simulink model "rate_limited_systems"  (R2021a)
settings: Solver=VariableStepAuto  StartTime=0.0  StopTime=10.0  RelTol=1e-3
settings Model: Creator=dimpa  LastModifiedBy=dimpa

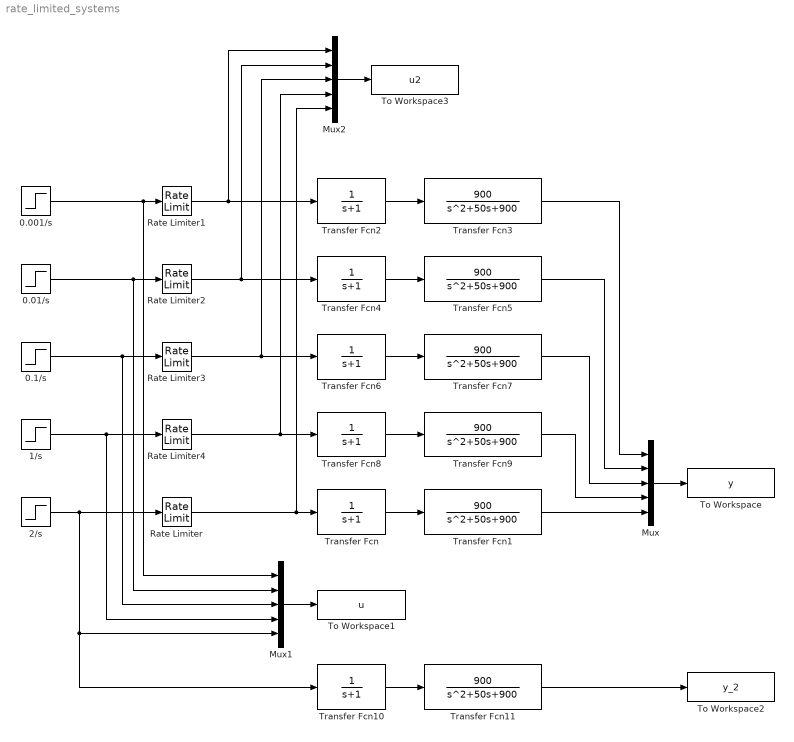
== system rate_limited_systems ==
  0.001/s : Step  After=0.001  SampleTime=0
  0.01/s : Step  After=0.01  SampleTime=0
  0.1/s : Step  After=0.1  SampleTime=0
  1/s : Step  SampleTime=0
  2/s : Step  After=2  SampleTime=0
  Mux : Mux  Inputs=5
  Mux1 : Mux  Inputs=5
  Mux2 : Mux  Inputs=5
  Rate Limiter{,1..4} (5 alike) : RateLimiter  RisingSlewLimit=0.3  SampleTimeMode=inherited
  To Workspace : ToWorkspace  VariableName=y  SaveFormat=Timeseries  SampleTime=-1
  To Workspace1 : ToWorkspace  VariableName=u  SaveFormat=Timeseries  SampleTime=-1
  To Workspace2 : ToWorkspace  VariableName=y_2  SaveFormat=Timeseries  SampleTime=-1
  To Workspace3 : ToWorkspace  VariableName=u2  SaveFormat=Timeseries  SampleTime=-1
  Transfer Fcn{,2,4,6,8,10} (6 alike) : TransferFcn  Denominator=[1 1]
  Transfer Fcn{1,3,5,7,9,11} (6 alike) : TransferFcn  Numerator=[900]  Denominator=[1 50 900]
  wires:
  0.001/s/1 -> Mux1/1, Rate Limiter1/1
  0.01/s/1 -> Mux1/2, Rate Limiter2/1
  0.1/s/1 -> Mux1/3, Rate Limiter3/1
  1/s/1 -> Mux1/4, Rate Limiter4/1
  2/s/1 -> Mux1/5, Transfer Fcn10/1, Rate Limiter/1
  Transfer Fcn/1 -> Transfer Fcn1/1
  Transfer Fcn1/1 -> Mux/5
  Transfer Fcn2/1 -> Transfer Fcn3/1
  Rate Limiter1/1 -> Transfer Fcn2/1, Mux2/1
  Rate Limiter2/1 -> Transfer Fcn4/1, Mux2/2
  Transfer Fcn4/1 -> Transfer Fcn5/1
  Transfer Fcn6/1 -> Transfer Fcn7/1
  Rate Limiter3/1 -> Transfer Fcn6/1, Mux2/3
  Rate Limiter4/1 -> Transfer Fcn8/1, Mux2/4
  Transfer Fcn8/1 -> Transfer Fcn9/1
  Transfer Fcn9/1 -> Mux/4
  Transfer Fcn7/1 -> Mux/3
  Transfer Fcn5/1 -> Mux/2
  Transfer Fcn3/1 -> Mux/1
  Mux/1 -> To Workspace/1
  Mux1/1 -> To Workspace1/1
  Transfer Fcn10/1 -> Transfer Fcn11/1
  Transfer Fcn11/1 -> To Workspace2/1
  Mux2/1 -> To Workspace3/1
  Rate Limiter/1 -> Transfer Fcn/1, Mux2/5
